simulink model "Alu8Bit"  (R2014a)
settings: Solver=ode45  StartTime=0.0  StopTime=10.0  RelTol=1e-3
libraries: hdlsllib x104
(part 1 of 5)
settings Model: Creator=you.r  LastModifiedBy=you.r
settings OptimizationCC: BlockReduction=off  ConditionallyExecuteInputs=off  InlineParams=on
settings DebuggingCC: AlgebraicLoopMsg=error
settings HardwareCC: ProdHWDeviceType=ASIC/FPGA->ASIC/FPGA  ProdEqTarget=off

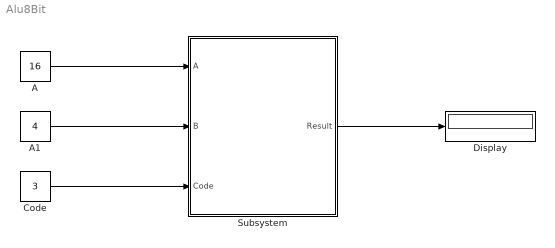
== system Alu8Bit ==
  A : Constant  Value=16  OutDataTypeStr=uint8  SampleTime=1
  A1 : Constant  Value=4  OutDataTypeStr=uint8  SampleTime=1
  Code : Constant  Value=3  OutDataTypeStr=uint8  SampleTime=1
  Display : Display
  Subsystem : Subsystem  TreatAsAtomicUnit=on
  wires:
  Subsystem/1(Result) -> Display/1
  A/1 -> Subsystem/1(A)
  A1/1 -> Subsystem/2(B)
  Code/1 -> Subsystem/3(Code)

== system Alu8Bit/Subsystem ==
  A : Inport  OutDataTypeStr=uint8  SampleTime=1
  B : Inport  Port=2  OutDataTypeStr=uint8  SampleTime=1
  Code : Inport  Port=3  OutDataTypeStr=uint8  SampleTime=1
  8-bit 4-to-1 MUX : Subsystem
  8-bit Adder : Subsystem
  8-bit Subtractor : Subsystem
  BitwiseAnd : Subsystem
  Multiplier : Subsystem
  Result : Outport
  wires:
  8-bit 4-to-1 MUX/1(y) -> Result/1
  BitwiseAnd/1(y) -> 8-bit 4-to-1 MUX/4(3)
  Multiplier/1(Out1) -> 8-bit 4-to-1 MUX/3(2)
  B/1 -> BitwiseAnd/2(b), Multiplier/2(In2), 8-bit Subtractor/2(In2), 8-bit Adder/2(In2)
  A/1 -> Multiplier/1(In1), BitwiseAnd/1(a), 8-bit Subtractor/1(In1), 8-bit Adder/1(In1)
  8-bit Subtractor/1(Out1) -> 8-bit 4-to-1 MUX/2(1)
  Code/1 -> 8-bit 4-to-1 MUX/5(C)
  8-bit Adder/1(Out1) -> 8-bit 4-to-1 MUX/1(0)

== system Alu8Bit/Subsystem/8-bit 4-to-1 MUX ==
  0 : Inport  OutDataTypeStr=uint8  SampleTime=1
  1 : Inport  Port=2  OutDataTypeStr=uint8  SampleTime=1
  2 : Inport  Port=3  OutDataTypeStr=uint8  SampleTime=1
  3 : Inport  Port=4  OutDataTypeStr=uint8  SampleTime=1
  C : Inport  Port=5  OutDataTypeStr=uint8  SampleTime=1
  Bit Concat : Subsystem
  Subsystem1 : Subsystem
  Subsystem2 : Subsystem
  Subsystem3 : Subsystem
  Subsystem4 : Subsystem
  Subsystem5 : Subsystem
  Subsystem6 : Subsystem
  Subsystem7 : Subsystem
  Subsystem8 : Subsystem
  X Slicer1 : Subsystem
  X Slicer2 : Subsystem
  X Slicer3 : Subsystem
  X Slicer4 : Subsystem
  X Slicer5 : Subsystem
  y : Outport  SampleTime=1
  wires:
  X Slicer1/4(Y3) -> Subsystem3/4(I2)
  1/1 -> X Slicer1/1(X)
  X Slicer3/2(Y1) -> Subsystem1/5(I3)
  X Slicer4/4(Y3) -> Subsystem3/6(I4)
  X Slicer1/1(Y0) -> Subsystem8/4(I2)
  X Slicer1/2(Y1) -> Subsystem1/4(I2)
  X Slicer2/3(Y2) -> Subsystem2/3(I1)
  X Slicer5/2(C2) -> Subsystem2/1(C2), Subsystem1/1(C2), Subsystem8/1(C2), Subsystem3/1(C2), Subsystem5/1(C2), Subsystem6/1(C2), Subsystem7/1(C2), Subsystem4/1(C2)
  X Slicer1/3(Y2) -> Subsystem2/4(I2)
  X Slicer3/7(Y6) -> Subsystem6/5(I3)
  X Slicer2/2(Y1) -> Subsystem1/3(I1)
  X Slicer5/1(C1) -> Subsystem2/2(C1), Subsystem1/2(C1), Subsystem8/2(C1), Subsystem3/2(C1), Subsystem4/2(C1), Subsystem5/2(C1), Subsystem7/2(C1), Subsystem6/2(C1)
  X Slicer4/1(Y0) -> Subsystem8/6(I4)
  0/1 -> X Slicer2/1(X)
  X Slicer3/1(Y0) -> Subsystem8/5(I3)
  X Slicer1/8(Y7) -> Subsystem7/4(I2)
  X Slicer1/5(Y4) -> Subsystem4/4(I2)
  X Slicer3/6(Y5) -> Subsystem5/5(I3)
  X Slicer4/2(Y1) -> Subsystem1/6(I4)
  X Slicer2/6(Y5) -> Subsystem5/3(I1)
  X Slicer4/6(Y5) -> Subsystem5/6(I4)
  X Slicer1/6(Y5) -> Subsystem5/4(I2)
  X Slicer2/1(Y0) -> Subsystem8/3(I1)
  X Slicer4/3(Y2) -> Subsystem2/6(I4)
  X Slicer2/5(Y4) -> Subsystem4/3(I1)
  2/1 -> X Slicer3/1(X)
  3/1 -> X Slicer4/1(X)
  X Slicer1/7(Y6) -> Subsystem6/4(I2)
  Bit Concat/1(Out1) -> y/1
  X Slicer4/7(Y6) -> Subsystem6/6(I4)
  X Slicer3/5(Y4) -> Subsystem4/5(I3)
  X Slicer2/7(Y6) -> Subsystem6/3(I1)
  C/1 -> X Slicer5/1(X)
  X Slicer2/4(Y3) -> Subsystem3/3(I1)
  X Slicer4/5(Y4) -> Subsystem4/6(I4)
  X Slicer3/4(Y3) -> Subsystem3/5(I3)
  X Slicer4/8(Y7) -> Subsystem7/6(I4)
  X Slicer3/8(Y7) -> Subsystem7/5(I3)
  Subsystem2/1(Out) -> Bit Concat/6(In6)
  Subsystem1/1(Out) -> Bit Concat/7(In7)
  Subsystem8/1(Out) -> Bit Concat/8(In8)
  Subsystem3/1(Out) -> Bit Concat/5(In5)
  Subsystem6/1(Out) -> Bit Concat/2(In2)
  Subsystem4/1(Out) -> Bit Concat/4(In4)
  Subsystem5/1(Out) -> Bit Concat/3(In3)
  Subsystem7/1(Out) -> Bit Concat/1(In1)
  X Slicer2/8(Y7) -> Subsystem7/3(I1)
  X Slicer3/3(Y2) -> Subsystem2/5(I3)

== system Alu8Bit/Subsystem/8-bit Adder ==
  In1 : Inport
  In2 : Inport  Port=2
  8-bit Adder : Subsystem
  Bit Concat : Subsystem
  Both Negative : Logic  AllPortsSameDT=off  OutDataTypeStr=boolean
  Both Positive : Logic  AllPortsSameDT=off  OutDataTypeStr=boolean
  "If both conditions true, overflow" : Logic  AllPortsSameDT=off  OutDataTypeStr=boolean
  "If both conditions true, overflow1" : Logic  AllPortsSameDT=off  OutDataTypeStr=boolean
  MSB Not High : Logic  Operator=NOT  AllPortsSameDT=off  OutDataTypeStr=boolean
  Negative Or MSB HIgh : Logic  Operator=XOR  AllPortsSameDT=off  OutDataTypeStr=boolean
  Positive A : Logic  Operator=NOT  AllPortsSameDT=off  OutDataTypeStr=boolean
  Positive B : Logic  Operator=NOT  AllPortsSameDT=off  OutDataTypeStr=boolean
  Positive or MSB not high : Logic  Operator=XOR  AllPortsSameDT=off  OutDataTypeStr=boolean
  Subtract : Constant  Value=0  OutDataTypeStr=boolean  SampleTime=1
  X Slicer : Subsystem
  X Slicer1 : Subsystem
  Xor : Logic  Operator=XOR  AllPortsSameDT=off  OutDataTypeStr=boolean
  Xor1 : Logic  Operator=XOR  AllPortsSameDT=off  OutDataTypeStr=boolean
  Out1 : Outport
  Out2 : Outport  Port=2
  wires:
  Bit Concat/1(Out1) -> Out1/1
  In1/1 -> X Slicer/1(X)
  In2/1 -> X Slicer1/1(X)
  8-bit Adder/8(Out8) -> Negative Or MSB HIgh/1, MSB Not High/1, Bit Concat/1(In1)
  8-bit Adder/7(Out7) -> Bit Concat/2(In2)
  8-bit Adder/6(Out6) -> Bit Concat/3(In3)
  8-bit Adder/5(Out5) -> Bit Concat/4(In4)
  8-bit Adder/4(Out4) -> Bit Concat/5(In5)
  8-bit Adder/3(Out3) -> Bit Concat/6(In6)
  8-bit Adder/2(Out2) -> Bit Concat/7(In7)
  8-bit Adder/1(Out1) -> Bit Concat/8(In8)
  X Slicer/1(Y0) -> 8-bit Adder/1(A1)
  X Slicer/2(Y1) -> 8-bit Adder/3(A2)
  X Slicer/3(Y2) -> 8-bit Adder/4(A3)
  X Slicer/4(Y3) -> 8-bit Adder/5(A4)
  X Slicer/5(Y4) -> 8-bit Adder/9(A5)
  X Slicer/6(Y5) -> 8-bit Adder/6(A6)
  X Slicer/7(Y6) -> 8-bit Adder/7(A7)
  X Slicer1/1(Y0) -> 8-bit Adder/2(B1)
  X Slicer1/2(Y1) -> 8-bit Adder/10(B2)
  X Slicer1/3(Y2) -> 8-bit Adder/11(B3)
  X Slicer1/4(Y3) -> 8-bit Adder/12(B4)
  X Slicer1/5(Y4) -> 8-bit Adder/16(B5)
  X Slicer1/6(Y5) -> 8-bit Adder/13(B6)
  X Slicer1/7(Y6) -> 8-bit Adder/14(B7)
  X Slicer1/8(Y7) -> Xor1/1, 8-bit Adder/15(B8)
  Both Negative/1 -> "If both conditions true, overflow"/2, Negative Or MSB HIgh/2
  Negative Or MSB HIgh/1 -> "If both conditions true, overflow"/1
  X Slicer/8(Y7) -> Positive A/1, Both Negative/1, 8-bit Adder/8(A8)
  Positive A/1 -> Both Positive/1
  Positive B/1 -> Both Positive/2
  Both Positive/1 -> "If both conditions true, overflow1"/1, Positive or MSB not high/1
  MSB Not High/1 -> Positive or MSB not high/2
  Positive or MSB not high/1 -> "If both conditions true, overflow1"/2
  Xor/1 -> Out2/1
  "If both conditions true, overflow1"/1 -> Xor/2
  "If both conditions true, overflow"/1 -> Xor/1
  Subtract/1 -> Xor1/2, 8-bit Adder/17(Subtraction?)
  Xor1/1 -> Positive B/1, Both Negative/2

== system Alu8Bit/Subsystem/8-bit Subtractor ==
  In1 : Inport
  In2 : Inport  Port=2
  8-bit Adder : Subsystem
  Bit Concat : Subsystem
  Both Negative : Logic  AllPortsSameDT=off  OutDataTypeStr=boolean
  Both Positive : Logic  AllPortsSameDT=off  OutDataTypeStr=boolean
  "If both conditions true, overflow" : Logic  AllPortsSameDT=off  OutDataTypeStr=boolean
  "If both conditions true, overflow1" : Logic  AllPortsSameDT=off  OutDataTypeStr=boolean
  MSB Not High : Logic  Operator=NOT  AllPortsSameDT=off  OutDataTypeStr=boolean
  Negative Or MSB HIgh : Logic  Operator=XOR  AllPortsSameDT=off  OutDataTypeStr=boolean
  Positive A : Logic  Operator=NOT  AllPortsSameDT=off  OutDataTypeStr=boolean
  Positive B : Logic  Operator=NOT  AllPortsSameDT=off  OutDataTypeStr=boolean
  Positive or MSB not high : Logic  Operator=XOR  AllPortsSameDT=off  OutDataTypeStr=boolean
  Subtract : Constant  OutDataTypeStr=boolean  SampleTime=1
  X Slicer : Subsystem
  X Slicer1 : Subsystem
  Xor : Logic  Operator=XOR  AllPortsSameDT=off  OutDataTypeStr=boolean
  Xor1 : Logic  Operator=XOR  AllPortsSameDT=off  OutDataTypeStr=boolean
  Out1 : Outport
  Out2 : Outport  Port=2
  wires:
  Bit Concat/1(Out1) -> Out1/1
  In1/1 -> X Slicer/1(X)
  In2/1 -> X Slicer1/1(X)
  8-bit Adder/8(Out8) -> Negative Or MSB HIgh/1, MSB Not High/1, Bit Concat/1(In1)
  8-bit Adder/7(Out7) -> Bit Concat/2(In2)
  8-bit Adder/6(Out6) -> Bit Concat/3(In3)
  8-bit Adder/5(Out5) -> Bit Concat/4(In4)
  8-bit Adder/4(Out4) -> Bit Concat/5(In5)
  8-bit Adder/3(Out3) -> Bit Concat/6(In6)
  8-bit Adder/2(Out2) -> Bit Concat/7(In7)
  8-bit Adder/1(Out1) -> Bit Concat/8(In8)
  X Slicer/1(Y0) -> 8-bit Adder/1(A1)
  X Slicer/2(Y1) -> 8-bit Adder/3(A2)
  X Slicer/3(Y2) -> 8-bit Adder/4(A3)
  X Slicer/4(Y3) -> 8-bit Adder/5(A4)
  X Slicer/5(Y4) -> 8-bit Adder/9(A5)
  X Slicer/6(Y5) -> 8-bit Adder/6(A6)
  X Slicer/7(Y6) -> 8-bit Adder/7(A7)
  X Slicer1/1(Y0) -> 8-bit Adder/2(B1)
  X Slicer1/2(Y1) -> 8-bit Adder/10(B2)
  X Slicer1/3(Y2) -> 8-bit Adder/11(B3)
  X Slicer1/4(Y3) -> 8-bit Adder/12(B4)
  X Slicer1/5(Y4) -> 8-bit Adder/16(B5)
  X Slicer1/6(Y5) -> 8-bit Adder/13(B6)
  X Slicer1/7(Y6) -> 8-bit Adder/14(B7)
  X Slicer1/8(Y7) -> Xor1/1, 8-bit Adder/15(B8)
  Both Negative/1 -> "If both conditions true, overflow"/2, Negative Or MSB HIgh/2
  Negative Or MSB HIgh/1 -> "If both conditions true, overflow"/1
  X Slicer/8(Y7) -> Positive A/1, Both Negative/1, 8-bit Adder/8(A8)
  Positive A/1 -> Both Positive/1
  Positive B/1 -> Both Positive/2
  Both Positive/1 -> "If both conditions true, overflow1"/1, Positive or MSB not high/1
  MSB Not High/1 -> Positive or MSB not high/2
  Positive or MSB not high/1 -> "If both conditions true, overflow1"/2
  Xor/1 -> Out2/1
  "If both conditions true, overflow1"/1 -> Xor/2
  "If both conditions true, overflow"/1 -> Xor/1
  Subtract/1 -> Xor1/2, 8-bit Adder/17(Subtraction?)
  Xor1/1 -> Positive B/1, Both Negative/2

== system Alu8Bit/Subsystem/BitwiseAnd ==
  a : Inport  OutDataTypeStr=uint8  SampleTime=1
  b : Inport  Port=2  OutDataTypeStr=uint8  SampleTime=1
  Bit Concat : Subsystem
  Logical Operator{,1..7} (8 alike) : Logic  IconShape=distinctive  AllPortsSameDT=off  OutDataTypeStr=boolean  SampleTime=1
  X Slicer1 : Subsystem
  X Slicer2 : Subsystem
  y : Outport  SampleTime=1
  wires:
  b/1 -> X Slicer1/1(X)
  a/1 -> X Slicer2/1(X)
  Logical Operator2/1 -> Bit Concat/6(In6)
  Logical Operator4/1 -> Bit Concat/4(In4)
  Logical Operator7/1 -> Bit Concat/1(In1)
  Logical Operator/1 -> Bit Concat/8(In8)
  Logical Operator1/1 -> Bit Concat/7(In7)
  Logical Operator6/1 -> Bit Concat/2(In2)
  Logical Operator5/1 -> Bit Concat/3(In3)
  Logical Operator3/1 -> Bit Concat/5(In5)
  X Slicer1/8(Y7) -> Logical Operator7/2
  X Slicer1/5(Y4) -> Logical Operator4/2
  X Slicer2/4(Y3) -> Logical Operator3/1
  X Slicer2/8(Y7) -> Logical Operator7/1
  X Slicer2/3(Y2) -> Logical Operator2/1
  X Slicer2/6(Y5) -> Logical Operator5/1
  X Slicer2/2(Y1) -> Logical Operator1/1
  X Slicer1/3(Y2) -> Logical Operator2/2
  X Slicer1/2(Y1) -> Logical Operator1/2
  X Slicer1/7(Y6) -> Logical Operator6/2
  X Slicer2/7(Y6) -> Logical Operator6/1
  X Slicer2/5(Y4) -> Logical Operator4/1
  X Slicer1/1(Y0) -> Logical Operator/2
  X Slicer2/1(Y0) -> Logical Operator/1
  X Slicer1/6(Y5) -> Logical Operator5/2
  X Slicer1/4(Y3) -> Logical Operator3/2
  Bit Concat/1(Out1) -> y/1

== system Alu8Bit/Subsystem/Multiplier ==
  In1 : Inport  OutDataTypeStr=uint8
  In2 : Inport  Port=2  OutDataTypeStr=uint8
  Bit Concat : Subsystem
  Multiplier : Subsystem
  X Slicer : Subsystem
  X Slicer1 : Subsystem
  Out1 : Outport
  wires:
  In2/1 -> X Slicer1/1(X)
  In1/1 -> X Slicer/1(X)
  Bit Concat/1(Out1) -> Out1/1
  Multiplier/1(P0) -> Bit Concat/16(In16)
  Multiplier/2(P1) -> Bit Concat/15(In15)
  Multiplier/3(P2) -> Bit Concat/14(In14)
  Multiplier/4(P3) -> Bit Concat/13(In13)
  Multiplier/5(P4) -> Bit Concat/12(In12)
  Multiplier/6(P5) -> Bit Concat/11(In11)
  Multiplier/7(P6) -> Bit Concat/10(In10)
  Multiplier/8(P7) -> Bit Concat/9(In9)
  Multiplier/9(P15) -> Bit Concat/1(In1)
  Multiplier/10(P14) -> Bit Concat/2(In2)
  Multiplier/11(P13) -> Bit Concat/3(In3)
  Multiplier/12(P12) -> Bit Concat/4(In4)
  Multiplier/13(P11) -> Bit Concat/5(In5)
  Multiplier/14(P10) -> Bit Concat/6(In6)
  Multiplier/15(P9) -> Bit Concat/7(In7)
  Multiplier/16(P8) -> Bit Concat/8(In8)
  X Slicer/1(Y0) -> Multiplier/8(A0)
  X Slicer/2(Y1) -> Multiplier/7(A1)
  X Slicer/3(Y2) -> Multiplier/6(A2)
  X Slicer/4(Y3) -> Multiplier/5(A3)
  X Slicer/5(Y4) -> Multiplier/4(A4)
  X Slicer/6(Y5) -> Multiplier/3(A5)
  X Slicer/7(Y6) -> Multiplier/2(A6)
  X Slicer/8(Y7) -> Multiplier/1(A7)
  X Slicer1/1(Y0) -> Multiplier/9(B0)
  X Slicer1/2(Y1) -> Multiplier/10(B1)
  X Slicer1/3(Y2) -> Multiplier/11(B2)
  X Slicer1/4(Y3) -> Multiplier/12(B3)
  X Slicer1/5(Y4) -> Multiplier/13(B4)
  X Slicer1/6(Y5) -> Multiplier/14(B5)
  X Slicer1/7(Y6) -> Multiplier/15(B6)
  X Slicer1/8(Y7) -> Multiplier/16(B7)

== system Alu8Bit/Subsystem/8-bit 4-to-1 MUX/Bit Concat ==
  In1 : Inport
  In2 : Inport  Port=2
  In3 : Inport  Port=3
  In4 : Inport  Port=4
  In5 : Inport  Port=5
  In6 : Inport  Port=6
  In7 : Inport  Port=7
  In8 : Inport  Port=8
  Bit Concat : hdlsllib/HDL Operations/Bit Concat  numInputs=8
  Data Type Conversion : DataTypeConversion  OutDataTypeStr=uint8
  Out1 : Outport
  wires:
  Data Type Conversion/1 -> Out1/1
  Bit Concat/1 -> Data Type Conversion/1
  In7/1 -> Bit Concat/7
  In1/1 -> Bit Concat/1
  In8/1 -> Bit Concat/8
  In6/1 -> Bit Concat/6
  In2/1 -> Bit Concat/2
  In5/1 -> Bit Concat/5
  In3/1 -> Bit Concat/3
  In4/1 -> Bit Concat/4

== system Alu8Bit/Subsystem/8-bit 4-to-1 MUX/Subsystem1 ==
  C2 : Inport
  C1 : Inport  Port=2
  I1 : Inport  Port=3
  I2 : Inport  Port=4
  I3 : Inport  Port=5
  I4 : Inport  Port=6
  Logical Operator{,1..5,7,9} (8 alike) : Logic  IconShape=distinctive  AllPortsSameDT=off  OutDataTypeStr=boolean
  Logical Operator10 : Logic  Operator=NOT  IconShape=distinctive  AllPortsSameDT=off  OutDataTypeStr=boolean
  Logical Operator6 : Logic  Operator=OR  Inputs=4  IconShape=distinctive  AllPortsSameDT=off  OutDataTypeStr=boolean
  Logical Operator8 : Logic  Operator=NOT  IconShape=distinctive  AllPortsSameDT=off  OutDataTypeStr=boolean
  Out : Outport
  wires:
  I1/1 -> Logical Operator2/1
  I3/1 -> Logical Operator5/1
  Logical Operator4/1 -> Logical Operator6/4
  Logical Operator3/1 -> Logical Operator6/2
  C1/1 -> Logical Operator10/1, Logical Operator/2, Logical Operator7/2
  C2/1 -> Logical Operator9/2, Logical Operator/1, Logical Operator8/1
  Logical Operator10/1 -> Logical Operator1/1, Logical Operator9/1
  Logical Operator/1 -> Logical Operator4/2
  Logical Operator7/1 -> Logical Operator3/2
  I2/1 -> Logical Operator3/1
  Logical Operator2/1 -> Logical Operator6/1
  Logical Operator9/1 -> Logical Operator5/2
  I4/1 -> Logical Operator4/1
  Logical Operator5/1 -> Logical Operator6/3
  Logical Operator6/1 -> Out/1
  Logical Operator8/1 -> Logical Operator1/2, Logical Operator7/1
  Logical Operator1/1 -> Logical Operator2/2

== system Alu8Bit/Subsystem/8-bit 4-to-1 MUX/Subsystem2 ==
  C2 : Inport
  C1 : Inport  Port=2
  I1 : Inport  Port=3
  I2 : Inport  Port=4
  I3 : Inport  Port=5
  I4 : Inport  Port=6
  Logical Operator{,1..5,7,9} (8 alike) : Logic  IconShape=distinctive  AllPortsSameDT=off  OutDataTypeStr=boolean
  Logical Operator10 : Logic  Operator=NOT  IconShape=distinctive  AllPortsSameDT=off  OutDataTypeStr=boolean
  Logical Operator6 : Logic  Operator=OR  Inputs=4  IconShape=distinctive  AllPortsSameDT=off  OutDataTypeStr=boolean
  Logical Operator8 : Logic  Operator=NOT  IconShape=distinctive  AllPortsSameDT=off  OutDataTypeStr=boolean
  Out : Outport
  wires:
  I1/1 -> Logical Operator2/1
  I3/1 -> Logical Operator5/1
  Logical Operator4/1 -> Logical Operator6/4
  Logical Operator3/1 -> Logical Operator6/2
  C1/1 -> Logical Operator10/1, Logical Operator/2, Logical Operator7/2
  C2/1 -> Logical Operator9/2, Logical Operator/1, Logical Operator8/1
  Logical Operator10/1 -> Logical Operator1/1, Logical Operator9/1
  Logical Operator/1 -> Logical Operator4/2
  Logical Operator7/1 -> Logical Operator3/2
  I2/1 -> Logical Operator3/1
  Logical Operator2/1 -> Logical Operator6/1
  Logical Operator9/1 -> Logical Operator5/2
  I4/1 -> Logical Operator4/1
  Logical Operator5/1 -> Logical Operator6/3
  Logical Operator6/1 -> Out/1
  Logical Operator8/1 -> Logical Operator1/2, Logical Operator7/1
  Logical Operator1/1 -> Logical Operator2/2

== system Alu8Bit/Subsystem/8-bit 4-to-1 MUX/Subsystem3 ==
  C2 : Inport
  C1 : Inport  Port=2
  I1 : Inport  Port=3
  I2 : Inport  Port=4
  I3 : Inport  Port=5
  I4 : Inport  Port=6
  Logical Operator{,1..5,7,9} (8 alike) : Logic  IconShape=distinctive  AllPortsSameDT=off  OutDataTypeStr=boolean
  Logical Operator10 : Logic  Operator=NOT  IconShape=distinctive  AllPortsSameDT=off  OutDataTypeStr=boolean
  Logical Operator6 : Logic  Operator=OR  Inputs=4  IconShape=distinctive  AllPortsSameDT=off  OutDataTypeStr=boolean
  Logical Operator8 : Logic  Operator=NOT  IconShape=distinctive  AllPortsSameDT=off  OutDataTypeStr=boolean
  Out : Outport
  wires:
  I1/1 -> Logical Operator2/1
  I3/1 -> Logical Operator5/1
  Logical Operator4/1 -> Logical Operator6/4
  Logical Operator3/1 -> Logical Operator6/2
  C1/1 -> Logical Operator10/1, Logical Operator/2, Logical Operator7/2
  C2/1 -> Logical Operator9/2, Logical Operator/1, Logical Operator8/1
  Logical Operator10/1 -> Logical Operator1/1, Logical Operator9/1
  Logical Operator/1 -> Logical Operator4/2
  Logical Operator7/1 -> Logical Operator3/2
  I2/1 -> Logical Operator3/1
  Logical Operator2/1 -> Logical Operator6/1
  Logical Operator9/1 -> Logical Operator5/2
  I4/1 -> Logical Operator4/1
  Logical Operator5/1 -> Logical Operator6/3
  Logical Operator6/1 -> Out/1
  Logical Operator8/1 -> Logical Operator1/2, Logical Operator7/1
  Logical Operator1/1 -> Logical Operator2/2

== system Alu8Bit/Subsystem/8-bit 4-to-1 MUX/Subsystem4 ==
  C2 : Inport
  C1 : Inport  Port=2
  I1 : Inport  Port=3
  I2 : Inport  Port=4
  I3 : Inport  Port=5
  I4 : Inport  Port=6
  Logical Operator{,1..5,7,9} (8 alike) : Logic  IconShape=distinctive  AllPortsSameDT=off  OutDataTypeStr=boolean
  Logical Operator10 : Logic  Operator=NOT  IconShape=distinctive  AllPortsSameDT=off  OutDataTypeStr=boolean
  Logical Operator6 : Logic  Operator=OR  Inputs=4  IconShape=distinctive  AllPortsSameDT=off  OutDataTypeStr=boolean
  Logical Operator8 : Logic  Operator=NOT  IconShape=distinctive  AllPortsSameDT=off  OutDataTypeStr=boolean
  Out : Outport
  wires:
  I1/1 -> Logical Operator2/1
  I3/1 -> Logical Operator5/1
  Logical Operator4/1 -> Logical Operator6/4
  Logical Operator3/1 -> Logical Operator6/2
  C1/1 -> Logical Operator10/1, Logical Operator/2, Logical Operator7/2
  C2/1 -> Logical Operator9/2, Logical Operator/1, Logical Operator8/1
  Logical Operator10/1 -> Logical Operator1/1, Logical Operator9/1
  Logical Operator/1 -> Logical Operator4/2
  Logical Operator7/1 -> Logical Operator3/2
  I2/1 -> Logical Operator3/1
  Logical Operator2/1 -> Logical Operator6/1
  Logical Operator9/1 -> Logical Operator5/2
  I4/1 -> Logical Operator4/1
  Logical Operator5/1 -> Logical Operator6/3
  Logical Operator6/1 -> Out/1
  Logical Operator8/1 -> Logical Operator1/2, Logical Operator7/1
  Logical Operator1/1 -> Logical Operator2/2

== system Alu8Bit/Subsystem/8-bit 4-to-1 MUX/Subsystem5 ==
  C2 : Inport
  C1 : Inport  Port=2
  I1 : Inport  Port=3
  I2 : Inport  Port=4
  I3 : Inport  Port=5
  I4 : Inport  Port=6
  Logical Operator{,1..5,7,9} (8 alike) : Logic  IconShape=distinctive  AllPortsSameDT=off  OutDataTypeStr=boolean
  Logical Operator10 : Logic  Operator=NOT  IconShape=distinctive  AllPortsSameDT=off  OutDataTypeStr=boolean
  Logical Operator6 : Logic  Operator=OR  Inputs=4  IconShape=distinctive  AllPortsSameDT=off  OutDataTypeStr=boolean
  Logical Operator8 : Logic  Operator=NOT  IconShape=distinctive  AllPortsSameDT=off  OutDataTypeStr=boolean
  Out : Outport
  wires:
  I1/1 -> Logical Operator2/1
  I3/1 -> Logical Operator5/1
  Logical Operator4/1 -> Logical Operator6/4
  Logical Operator3/1 -> Logical Operator6/2
  C1/1 -> Logical Operator10/1, Logical Operator/2, Logical Operator7/2
  C2/1 -> Logical Operator9/2, Logical Operator/1, Logical Operator8/1
  Logical Operator10/1 -> Logical Operator1/1, Logical Operator9/1
  Logical Operator/1 -> Logical Operator4/2
  Logical Operator7/1 -> Logical Operator3/2
  I2/1 -> Logical Operator3/1
  Logical Operator2/1 -> Logical Operator6/1
  Logical Operator9/1 -> Logical Operator5/2
  I4/1 -> Logical Operator4/1
  Logical Operator5/1 -> Logical Operator6/3
  Logical Operator6/1 -> Out/1
  Logical Operator8/1 -> Logical Operator1/2, Logical Operator7/1
  Logical Operator1/1 -> Logical Operator2/2

== system Alu8Bit/Subsystem/8-bit 4-to-1 MUX/Subsystem6 ==
  C2 : Inport
  C1 : Inport  Port=2
  I1 : Inport  Port=3
  I2 : Inport  Port=4
  I3 : Inport  Port=5
  I4 : Inport  Port=6
  Logical Operator{,1..5,7,9} (8 alike) : Logic  IconShape=distinctive  AllPortsSameDT=off  OutDataTypeStr=boolean
  Logical Operator10 : Logic  Operator=NOT  IconShape=distinctive  AllPortsSameDT=off  OutDataTypeStr=boolean
  Logical Operator6 : Logic  Operator=OR  Inputs=4  IconShape=distinctive  AllPortsSameDT=off  OutDataTypeStr=boolean
  Logical Operator8 : Logic  Operator=NOT  IconShape=distinctive  AllPortsSameDT=off  OutDataTypeStr=boolean
  Out : Outport
  wires:
  I1/1 -> Logical Operator2/1
  I3/1 -> Logical Operator5/1
  Logical Operator4/1 -> Logical Operator6/4
  Logical Operator3/1 -> Logical Operator6/2
  C1/1 -> Logical Operator10/1, Logical Operator/2, Logical Operator7/2
  C2/1 -> Logical Operator9/2, Logical Operator/1, Logical Operator8/1
  Logical Operator10/1 -> Logical Operator1/1, Logical Operator9/1
  Logical Operator/1 -> Logical Operator4/2
  Logical Operator7/1 -> Logical Operator3/2
  I2/1 -> Logical Operator3/1
  Logical Operator2/1 -> Logical Operator6/1
  Logical Operator9/1 -> Logical Operator5/2
  I4/1 -> Logical Operator4/1
  Logical Operator5/1 -> Logical Operator6/3
  Logical Operator6/1 -> Out/1
  Logical Operator8/1 -> Logical Operator1/2, Logical Operator7/1
  Logical Operator1/1 -> Logical Operator2/2

== system Alu8Bit/Subsystem/8-bit 4-to-1 MUX/Subsystem7 ==
  C2 : Inport
  C1 : Inport  Port=2
  I1 : Inport  Port=3
  I2 : Inport  Port=4
  I3 : Inport  Port=5
  I4 : Inport  Port=6
  Logical Operator{,1..5,7,9} (8 alike) : Logic  IconShape=distinctive  AllPortsSameDT=off  OutDataTypeStr=boolean
  Logical Operator10 : Logic  Operator=NOT  IconShape=distinctive  AllPortsSameDT=off  OutDataTypeStr=boolean
  Logical Operator6 : Logic  Operator=OR  Inputs=4  IconShape=distinctive  AllPortsSameDT=off  OutDataTypeStr=boolean
  Logical Operator8 : Logic  Operator=NOT  IconShape=distinctive  AllPortsSameDT=off  OutDataTypeStr=boolean
  Out : Outport
  wires:
  I1/1 -> Logical Operator2/1
  I3/1 -> Logical Operator5/1
  Logical Operator4/1 -> Logical Operator6/4
  Logical Operator3/1 -> Logical Operator6/2
  C1/1 -> Logical Operator10/1, Logical Operator/2, Logical Operator7/2
  C2/1 -> Logical Operator9/2, Logical Operator/1, Logical Operator8/1
  Logical Operator10/1 -> Logical Operator1/1, Logical Operator9/1
  Logical Operator/1 -> Logical Operator4/2
  Logical Operator7/1 -> Logical Operator3/2
  I2/1 -> Logical Operator3/1
  Logical Operator2/1 -> Logical Operator6/1
  Logical Operator9/1 -> Logical Operator5/2
  I4/1 -> Logical Operator4/1
  Logical Operator5/1 -> Logical Operator6/3
  Logical Operator6/1 -> Out/1
  Logical Operator8/1 -> Logical Operator1/2, Logical Operator7/1
  Logical Operator1/1 -> Logical Operator2/2

== system Alu8Bit/Subsystem/8-bit 4-to-1 MUX/Subsystem8 ==
  C2 : Inport
  C1 : Inport  Port=2
  I1 : Inport  Port=3
  I2 : Inport  Port=4
  I3 : Inport  Port=5
  I4 : Inport  Port=6
  Logical Operator{,1..5,7,9} (8 alike) : Logic  IconShape=distinctive  AllPortsSameDT=off  OutDataTypeStr=boolean
  Logical Operator10 : Logic  Operator=NOT  IconShape=distinctive  AllPortsSameDT=off  OutDataTypeStr=boolean
  Logical Operator6 : Logic  Operator=OR  Inputs=4  IconShape=distinctive  AllPortsSameDT=off  OutDataTypeStr=boolean
  Logical Operator8 : Logic  Operator=NOT  IconShape=distinctive  AllPortsSameDT=off  OutDataTypeStr=boolean
  Out : Outport
  wires:
  I1/1 -> Logical Operator2/1
  I3/1 -> Logical Operator5/1
  Logical Operator4/1 -> Logical Operator6/4
  Logical Operator3/1 -> Logical Operator6/2
  C1/1 -> Logical Operator10/1, Logical Operator/2, Logical Operator7/2
  C2/1 -> Logical Operator9/2, Logical Operator/1, Logical Operator8/1
  Logical Operator10/1 -> Logical Operator1/1, Logical Operator9/1
  Logical Operator/1 -> Logical Operator4/2
  Logical Operator7/1 -> Logical Operator3/2
  I2/1 -> Logical Operator3/1
  Logical Operator2/1 -> Logical Operator6/1
  Logical Operator9/1 -> Logical Operator5/2
  I4/1 -> Logical Operator4/1
  Logical Operator5/1 -> Logical Operator6/3
  Logical Operator6/1 -> Out/1
  Logical Operator8/1 -> Logical Operator1/2, Logical Operator7/1
  Logical Operator1/1 -> Logical Operator2/2

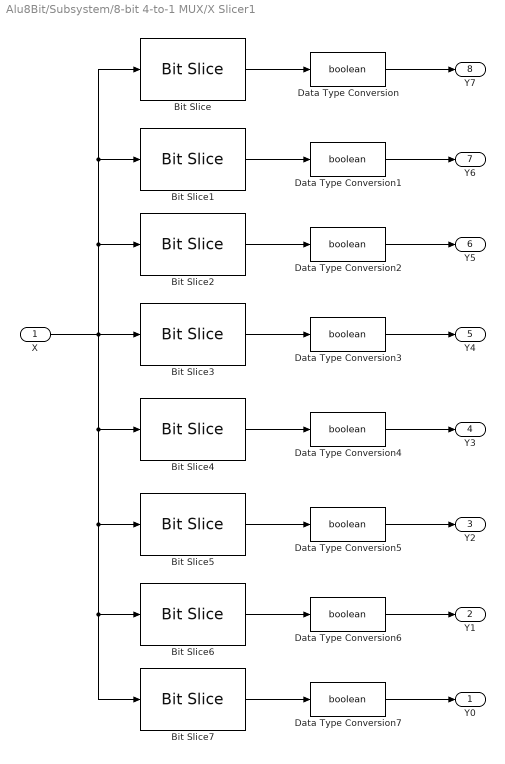
== system Alu8Bit/Subsystem/8-bit 4-to-1 MUX/X Slicer1 ==
  X : Inport  OutDataTypeStr=uint8  SampleTime=1
  Bit Slice : hdlsllib/HDL Operations/Bit Slice  lidx=7  ridx=7
  Bit Slice1 : hdlsllib/HDL Operations/Bit Slice  lidx=6  ridx=6
  Bit Slice2 : hdlsllib/HDL Operations/Bit Slice  lidx=5  ridx=5
  Bit Slice3 : hdlsllib/HDL Operations/Bit Slice  lidx=4  ridx=4
  Bit Slice4 : hdlsllib/HDL Operations/Bit Slice  lidx=3  ridx=3
  Bit Slice5 : hdlsllib/HDL Operations/Bit Slice  lidx=2  ridx=2
  Bit Slice6 : hdlsllib/HDL Operations/Bit Slice  lidx=1  ridx=1
  Bit Slice7 : hdlsllib/HDL Operations/Bit Slice  lidx=0  ridx=0
  Data Type Conversion{,1..7} (8 alike) : DataTypeConversion  OutDataTypeStr=boolean
  Y0 : Outport  OutDataTypeStr=boolean  SampleTime=1
  Y1 : Outport  Port=2  OutDataTypeStr=boolean  SampleTime=1
  Y2 : Outport  Port=3  OutDataTypeStr=boolean  SampleTime=1
  Y3 : Outport  Port=4  OutDataTypeStr=boolean  SampleTime=1
  Y4 : Outport  Port=5  OutDataTypeStr=boolean  SampleTime=1
  Y5 : Outport  Port=6  OutDataTypeStr=boolean  SampleTime=1
  Y6 : Outport  Port=7  OutDataTypeStr=boolean  SampleTime=1
  Y7 : Outport  Port=8  OutDataTypeStr=boolean  SampleTime=1
  wires:
  X/1 -> Bit Slice4/1, Bit Slice5/1, Bit Slice6/1, Bit Slice7/1, Bit Slice3/1, Bit Slice2/1, Bit Slice1/1, Bit Slice/1
  Data Type Conversion/1 -> Y7/1
  Data Type Conversion1/1 -> Y6/1
  Bit Slice2/1 -> Data Type Conversion2/1
  Bit Slice3/1 -> Data Type Conversion3/1
  Bit Slice4/1 -> Data Type Conversion4/1
  Data Type Conversion6/1 -> Y1/1
  Bit Slice/1 -> Data Type Conversion/1
  Bit Slice1/1 -> Data Type Conversion1/1
  Bit Slice6/1 -> Data Type Conversion6/1
  Data Type Conversion7/1 -> Y0/1
  Bit Slice7/1 -> Data Type Conversion7/1
  Bit Slice5/1 -> Data Type Conversion5/1
  Data Type Conversion2/1 -> Y5/1
  Data Type Conversion3/1 -> Y4/1
  Data Type Conversion4/1 -> Y3/1
  Data Type Conversion5/1 -> Y2/1

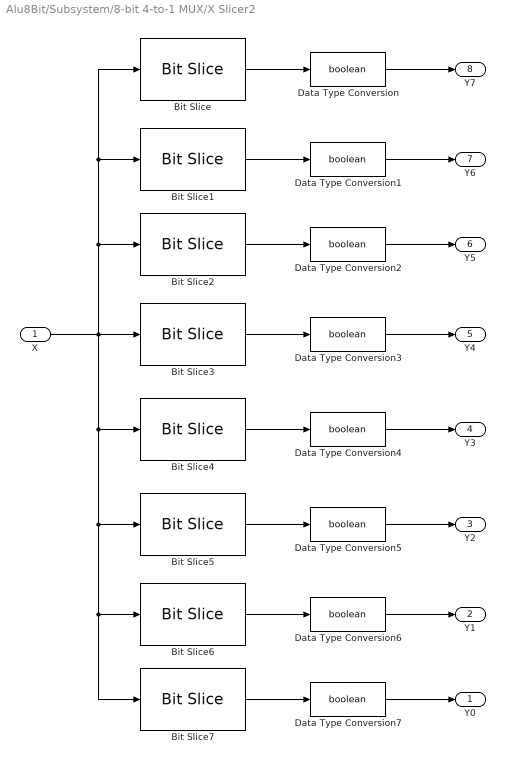
== system Alu8Bit/Subsystem/8-bit 4-to-1 MUX/X Slicer2 ==
  X : Inport  OutDataTypeStr=uint8  SampleTime=1
  Bit Slice : hdlsllib/HDL Operations/Bit Slice  lidx=7  ridx=7
  Bit Slice1 : hdlsllib/HDL Operations/Bit Slice  lidx=6  ridx=6
  Bit Slice2 : hdlsllib/HDL Operations/Bit Slice  lidx=5  ridx=5
  Bit Slice3 : hdlsllib/HDL Operations/Bit Slice  lidx=4  ridx=4
  Bit Slice4 : hdlsllib/HDL Operations/Bit Slice  lidx=3  ridx=3
  Bit Slice5 : hdlsllib/HDL Operations/Bit Slice  lidx=2  ridx=2
  Bit Slice6 : hdlsllib/HDL Operations/Bit Slice  lidx=1  ridx=1
  Bit Slice7 : hdlsllib/HDL Operations/Bit Slice  lidx=0  ridx=0
  Data Type Conversion{,1..7} (8 alike) : DataTypeConversion  OutDataTypeStr=boolean
  Y0 : Outport  OutDataTypeStr=boolean  SampleTime=1
  Y1 : Outport  Port=2  OutDataTypeStr=boolean  SampleTime=1
  Y2 : Outport  Port=3  OutDataTypeStr=boolean  SampleTime=1
  Y3 : Outport  Port=4  OutDataTypeStr=boolean  SampleTime=1
  Y4 : Outport  Port=5  OutDataTypeStr=boolean  SampleTime=1
  Y5 : Outport  Port=6  OutDataTypeStr=boolean  SampleTime=1
  Y6 : Outport  Port=7  OutDataTypeStr=boolean  SampleTime=1
  Y7 : Outport  Port=8  OutDataTypeStr=boolean  SampleTime=1
  wires:
  X/1 -> Bit Slice4/1, Bit Slice5/1, Bit Slice6/1, Bit Slice7/1, Bit Slice3/1, Bit Slice2/1, Bit Slice1/1, Bit Slice/1
  Data Type Conversion/1 -> Y7/1
  Data Type Conversion1/1 -> Y6/1
  Bit Slice2/1 -> Data Type Conversion2/1
  Bit Slice3/1 -> Data Type Conversion3/1
  Bit Slice4/1 -> Data Type Conversion4/1
  Data Type Conversion6/1 -> Y1/1
  Bit Slice/1 -> Data Type Conversion/1
  Bit Slice1/1 -> Data Type Conversion1/1
  Bit Slice6/1 -> Data Type Conversion6/1
  Data Type Conversion7/1 -> Y0/1
  Bit Slice7/1 -> Data Type Conversion7/1
  Bit Slice5/1 -> Data Type Conversion5/1
  Data Type Conversion2/1 -> Y5/1
  Data Type Conversion3/1 -> Y4/1
  Data Type Conversion4/1 -> Y3/1
  Data Type Conversion5/1 -> Y2/1

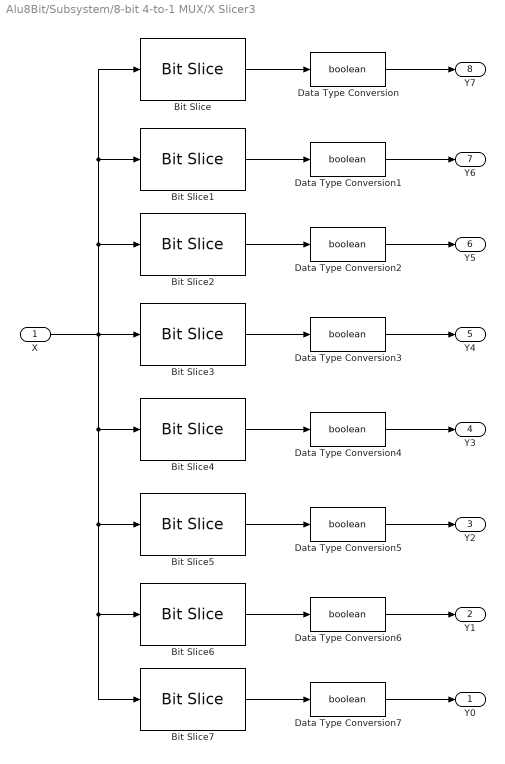
== system Alu8Bit/Subsystem/8-bit 4-to-1 MUX/X Slicer3 ==
  X : Inport  OutDataTypeStr=uint8  SampleTime=1
  Bit Slice : hdlsllib/HDL Operations/Bit Slice  lidx=7  ridx=7
  Bit Slice1 : hdlsllib/HDL Operations/Bit Slice  lidx=6  ridx=6
  Bit Slice2 : hdlsllib/HDL Operations/Bit Slice  lidx=5  ridx=5
  Bit Slice3 : hdlsllib/HDL Operations/Bit Slice  lidx=4  ridx=4
  Bit Slice4 : hdlsllib/HDL Operations/Bit Slice  lidx=3  ridx=3
  Bit Slice5 : hdlsllib/HDL Operations/Bit Slice  lidx=2  ridx=2
  Bit Slice6 : hdlsllib/HDL Operations/Bit Slice  lidx=1  ridx=1
  Bit Slice7 : hdlsllib/HDL Operations/Bit Slice  lidx=0  ridx=0
  Data Type Conversion{,1..7} (8 alike) : DataTypeConversion  OutDataTypeStr=boolean
  Y0 : Outport  OutDataTypeStr=boolean  SampleTime=1
  Y1 : Outport  Port=2  OutDataTypeStr=boolean  SampleTime=1
  Y2 : Outport  Port=3  OutDataTypeStr=boolean  SampleTime=1
  Y3 : Outport  Port=4  OutDataTypeStr=boolean  SampleTime=1
  Y4 : Outport  Port=5  OutDataTypeStr=boolean  SampleTime=1
  Y5 : Outport  Port=6  OutDataTypeStr=boolean  SampleTime=1
  Y6 : Outport  Port=7  OutDataTypeStr=boolean  SampleTime=1
  Y7 : Outport  Port=8  OutDataTypeStr=boolean  SampleTime=1
  wires:
  X/1 -> Bit Slice4/1, Bit Slice5/1, Bit Slice6/1, Bit Slice7/1, Bit Slice3/1, Bit Slice2/1, Bit Slice1/1, Bit Slice/1
  Data Type Conversion/1 -> Y7/1
  Data Type Conversion1/1 -> Y6/1
  Bit Slice2/1 -> Data Type Conversion2/1
  Bit Slice3/1 -> Data Type Conversion3/1
  Bit Slice4/1 -> Data Type Conversion4/1
  Data Type Conversion6/1 -> Y1/1
  Bit Slice/1 -> Data Type Conversion/1
  Bit Slice1/1 -> Data Type Conversion1/1
  Bit Slice6/1 -> Data Type Conversion6/1
  Data Type Conversion7/1 -> Y0/1
  Bit Slice7/1 -> Data Type Conversion7/1
  Bit Slice5/1 -> Data Type Conversion5/1
  Data Type Conversion2/1 -> Y5/1
  Data Type Conversion3/1 -> Y4/1
  Data Type Conversion4/1 -> Y3/1
  Data Type Conversion5/1 -> Y2/1

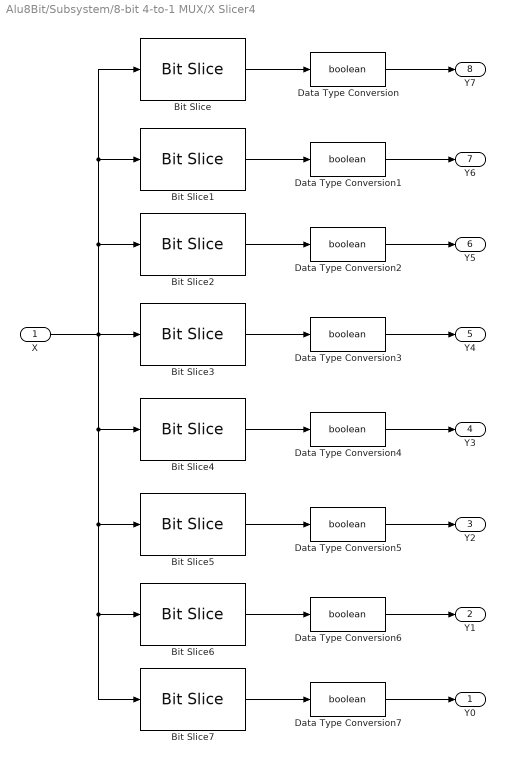
== system Alu8Bit/Subsystem/8-bit 4-to-1 MUX/X Slicer4 ==
  X : Inport  OutDataTypeStr=uint8  SampleTime=1
  Bit Slice : hdlsllib/HDL Operations/Bit Slice  lidx=7  ridx=7
  Bit Slice1 : hdlsllib/HDL Operations/Bit Slice  lidx=6  ridx=6
  Bit Slice2 : hdlsllib/HDL Operations/Bit Slice  lidx=5  ridx=5
  Bit Slice3 : hdlsllib/HDL Operations/Bit Slice  lidx=4  ridx=4
  Bit Slice4 : hdlsllib/HDL Operations/Bit Slice  lidx=3  ridx=3
  Bit Slice5 : hdlsllib/HDL Operations/Bit Slice  lidx=2  ridx=2
  Bit Slice6 : hdlsllib/HDL Operations/Bit Slice  lidx=1  ridx=1
  Bit Slice7 : hdlsllib/HDL Operations/Bit Slice  lidx=0  ridx=0
  Data Type Conversion{,1..7} (8 alike) : DataTypeConversion  OutDataTypeStr=boolean
  Y0 : Outport  OutDataTypeStr=boolean  SampleTime=1
  Y1 : Outport  Port=2  OutDataTypeStr=boolean  SampleTime=1
  Y2 : Outport  Port=3  OutDataTypeStr=boolean  SampleTime=1
  Y3 : Outport  Port=4  OutDataTypeStr=boolean  SampleTime=1
  Y4 : Outport  Port=5  OutDataTypeStr=boolean  SampleTime=1
  Y5 : Outport  Port=6  OutDataTypeStr=boolean  SampleTime=1
  Y6 : Outport  Port=7  OutDataTypeStr=boolean  SampleTime=1
  Y7 : Outport  Port=8  OutDataTypeStr=boolean  SampleTime=1
  wires:
  X/1 -> Bit Slice4/1, Bit Slice5/1, Bit Slice6/1, Bit Slice7/1, Bit Slice3/1, Bit Slice2/1, Bit Slice1/1, Bit Slice/1
  Data Type Conversion/1 -> Y7/1
  Data Type Conversion1/1 -> Y6/1
  Bit Slice2/1 -> Data Type Conversion2/1
  Bit Slice3/1 -> Data Type Conversion3/1
  Bit Slice4/1 -> Data Type Conversion4/1
  Data Type Conversion6/1 -> Y1/1
  Bit Slice/1 -> Data Type Conversion/1
  Bit Slice1/1 -> Data Type Conversion1/1
  Bit Slice6/1 -> Data Type Conversion6/1
  Data Type Conversion7/1 -> Y0/1
  Bit Slice7/1 -> Data Type Conversion7/1
  Bit Slice5/1 -> Data Type Conversion5/1
  Data Type Conversion2/1 -> Y5/1
  Data Type Conversion3/1 -> Y4/1
  Data Type Conversion4/1 -> Y3/1
  Data Type Conversion5/1 -> Y2/1

== system Alu8Bit/Subsystem/8-bit 4-to-1 MUX/X Slicer5 ==
  X : Inport  OutDataTypeStr=uint8  SampleTime=1
  Bit Slice6 : hdlsllib/HDL Operations/Bit Slice  lidx=1  ridx=1
  Bit Slice7 : hdlsllib/HDL Operations/Bit Slice  lidx=0  ridx=0
  Data Type Conversion6 : DataTypeConversion  OutDataTypeStr=boolean
  Data Type Conversion7 : DataTypeConversion  OutDataTypeStr=boolean
  C1 : Outport  OutDataTypeStr=boolean  SampleTime=1
  C2 : Outport  Port=2  OutDataTypeStr=boolean  SampleTime=1
  wires:
  X/1 -> Bit Slice6/1, Bit Slice7/1
  Data Type Conversion6/1 -> C2/1
  Bit Slice6/1 -> Data Type Conversion6/1
  Data Type Conversion7/1 -> C1/1
  Bit Slice7/1 -> Data Type Conversion7/1

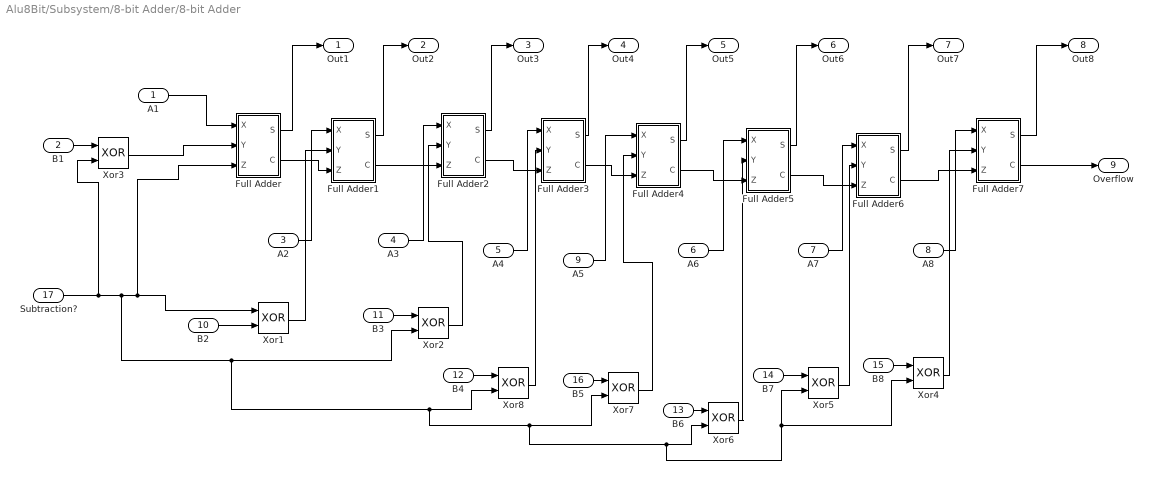
== system Alu8Bit/Subsystem/8-bit Adder/8-bit Adder ==
  A1 : Inport
  B1 : Inport  Port=2
  A2 : Inport  Port=3
  A3 : Inport  Port=4
  A4 : Inport  Port=5
  A6 : Inport  Port=6
  A7 : Inport  Port=7
  A8 : Inport  Port=8
  A5 : Inport  Port=9
  B2 : Inport  Port=10
  B3 : Inport  Port=11
  B4 : Inport  Port=12
  B6 : Inport  Port=13
  B7 : Inport  Port=14
  B8 : Inport  Port=15
  B5 : Inport  Port=16
  Subtraction? : Inport  Port=17  OutDataTypeStr=boolean
  Full Adder : Subsystem
  Full Adder1 : Subsystem
  Full Adder2 : Subsystem
  Full Adder3 : Subsystem
  Full Adder4 : Subsystem
  Full Adder5 : Subsystem
  Full Adder6 : Subsystem
  Full Adder7 : Subsystem
  Xor{1..8} (8 alike) : Logic  Operator=XOR  AllPortsSameDT=off  OutDataTypeStr=boolean
  Out1 : Outport  OutDataTypeStr=boolean
  Out2 : Outport  Port=2  OutDataTypeStr=boolean
  Out3 : Outport  Port=3  OutDataTypeStr=boolean
  Out4 : Outport  Port=4  OutDataTypeStr=boolean
  Out5 : Outport  Port=5  OutDataTypeStr=boolean
  Out6 : Outport  Port=6  OutDataTypeStr=boolean
  Out7 : Outport  Port=7  OutDataTypeStr=boolean
  Out8 : Outport  Port=8  OutDataTypeStr=boolean
  Overflow : Outport  Port=9  OutDataTypeStr=boolean
  wires:
  Full Adder7/2(C) -> Overflow/1
  Full Adder5/2(C) -> Full Adder6/3(Z)
  Full Adder7/1(S) -> Out8/1
  Full Adder4/2(C) -> Full Adder5/3(Z)
  Full Adder/2(C) -> Full Adder1/3(Z)
  Full Adder6/2(C) -> Full Adder7/3(Z)
  Full Adder6/1(S) -> Out7/1
  Full Adder2/2(C) -> Full Adder3/3(Z)
  Full Adder4/1(S) -> Out5/1
  A2/1 -> Full Adder1/1(X)
  A5/1 -> Full Adder4/1(X)
  Full Adder1/1(S) -> Out2/1
  A7/1 -> Full Adder6/1(X)
  Full Adder5/1(S) -> Out6/1
  A1/1 -> Full Adder/1(X)
  A8/1 -> Full Adder7/1(X)
  A6/1 -> Full Adder5/1(X)
  A4/1 -> Full Adder3/1(X)
  Full Adder3/1(S) -> Out4/1
  Full Adder/1(S) -> Out1/1
  Full Adder1/2(C) -> Full Adder2/3(Z)
  A3/1 -> Full Adder2/1(X)
  Full Adder3/2(C) -> Full Adder4/3(Z)
  Full Adder2/1(S) -> Out3/1
  B2/1 -> Xor1/2
  Subtraction?/1 -> Xor3/2, Xor4/2, Xor5/2, Xor6/2, Xor7/2, Xor8/2, Xor2/2, Full Adder/3(Z), Xor1/1
  Xor1/1 -> Full Adder1/2(Y)
  Xor2/1 -> Full Adder2/2(Y)
  B3/1 -> Xor2/1
  B4/1 -> Xor8/1
  Xor8/1 -> Full Adder3/2(Y)
  B5/1 -> Xor7/1
  Xor7/1 -> Full Adder4/2(Y)
  B6/1 -> Xor6/1
  Xor6/1 -> Full Adder5/2(Y)
  B7/1 -> Xor5/1
  Xor5/1 -> Full Adder6/2(Y)
  Xor4/1 -> Full Adder7/2(Y)
  B8/1 -> Xor4/1
  Xor3/1 -> Full Adder/2(Y)
  B1/1 -> Xor3/1

== system Alu8Bit/Subsystem/8-bit Adder/Bit Concat ==
  In1 : Inport
  In2 : Inport  Port=2
  In3 : Inport  Port=3
  In4 : Inport  Port=4
  In5 : Inport  Port=5
  In6 : Inport  Port=6
  In7 : Inport  Port=7
  In8 : Inport  Port=8
  Bit Concat : hdlsllib/HDL Operations/Bit Concat  numInputs=8
  Data Type Conversion : DataTypeConversion  OutDataTypeStr=uint8
  Out1 : Outport
  wires:
  Data Type Conversion/1 -> Out1/1
  In1/1 -> Bit Concat/1
  In4/1 -> Bit Concat/4
  In2/1 -> Bit Concat/2
  In3/1 -> Bit Concat/3
  In5/1 -> Bit Concat/5
  In6/1 -> Bit Concat/6
  In7/1 -> Bit Concat/7
  In8/1 -> Bit Concat/8
  Bit Concat/1 -> Data Type Conversion/1

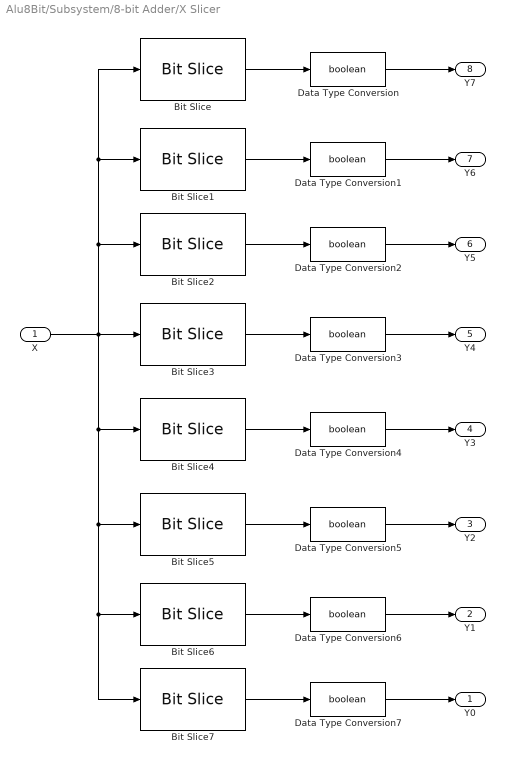
== system Alu8Bit/Subsystem/8-bit Adder/X Slicer ==
  X : Inport  OutDataTypeStr=uint8  SampleTime=1
  Bit Slice : hdlsllib/HDL Operations/Bit Slice  lidx=7  ridx=7
  Bit Slice1 : hdlsllib/HDL Operations/Bit Slice  lidx=6  ridx=6
  Bit Slice2 : hdlsllib/HDL Operations/Bit Slice  lidx=5  ridx=5
  Bit Slice3 : hdlsllib/HDL Operations/Bit Slice  lidx=4  ridx=4
  Bit Slice4 : hdlsllib/HDL Operations/Bit Slice  lidx=3  ridx=3
  Bit Slice5 : hdlsllib/HDL Operations/Bit Slice  lidx=2  ridx=2
  Bit Slice6 : hdlsllib/HDL Operations/Bit Slice  lidx=1  ridx=1
  Bit Slice7 : hdlsllib/HDL Operations/Bit Slice  lidx=0  ridx=0
  Data Type Conversion{,1..7} (8 alike) : DataTypeConversion  OutDataTypeStr=boolean
  Y0 : Outport
  Y1 : Outport  Port=2
  Y2 : Outport  Port=3
  Y3 : Outport  Port=4
  Y4 : Outport  Port=5
  Y5 : Outport  Port=6
  Y6 : Outport  Port=7
  Y7 : Outport  Port=8
  wires:
  X/1 -> Bit Slice4/1, Bit Slice5/1, Bit Slice6/1, Bit Slice7/1, Bit Slice3/1, Bit Slice2/1, Bit Slice1/1, Bit Slice/1
  Data Type Conversion/1 -> Y7/1
  Data Type Conversion1/1 -> Y6/1
  Bit Slice2/1 -> Data Type Conversion2/1
  Bit Slice3/1 -> Data Type Conversion3/1
  Bit Slice4/1 -> Data Type Conversion4/1
  Data Type Conversion6/1 -> Y1/1
  Bit Slice/1 -> Data Type Conversion/1
  Bit Slice1/1 -> Data Type Conversion1/1
  Bit Slice6/1 -> Data Type Conversion6/1
  Data Type Conversion7/1 -> Y0/1
  Bit Slice7/1 -> Data Type Conversion7/1
  Bit Slice5/1 -> Data Type Conversion5/1
  Data Type Conversion2/1 -> Y5/1
  Data Type Conversion3/1 -> Y4/1
  Data Type Conversion4/1 -> Y3/1
  Data Type Conversion5/1 -> Y2/1

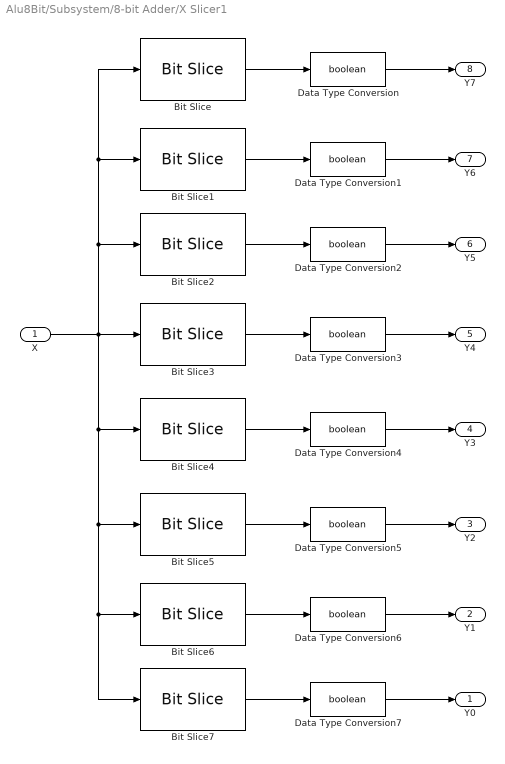
== system Alu8Bit/Subsystem/8-bit Adder/X Slicer1 ==
  X : Inport  OutDataTypeStr=uint8  SampleTime=1
  Bit Slice : hdlsllib/HDL Operations/Bit Slice  lidx=7  ridx=7
  Bit Slice1 : hdlsllib/HDL Operations/Bit Slice  lidx=6  ridx=6
  Bit Slice2 : hdlsllib/HDL Operations/Bit Slice  lidx=5  ridx=5
  Bit Slice3 : hdlsllib/HDL Operations/Bit Slice  lidx=4  ridx=4
  Bit Slice4 : hdlsllib/HDL Operations/Bit Slice  lidx=3  ridx=3
  Bit Slice5 : hdlsllib/HDL Operations/Bit Slice  lidx=2  ridx=2
  Bit Slice6 : hdlsllib/HDL Operations/Bit Slice  lidx=1  ridx=1
  Bit Slice7 : hdlsllib/HDL Operations/Bit Slice  lidx=0  ridx=0
  Data Type Conversion{,1..7} (8 alike) : DataTypeConversion  OutDataTypeStr=boolean
  Y0 : Outport
  Y1 : Outport  Port=2
  Y2 : Outport  Port=3
  Y3 : Outport  Port=4
  Y4 : Outport  Port=5
  Y5 : Outport  Port=6
  Y6 : Outport  Port=7
  Y7 : Outport  Port=8
  wires:
  X/1 -> Bit Slice4/1, Bit Slice5/1, Bit Slice6/1, Bit Slice7/1, Bit Slice3/1, Bit Slice2/1, Bit Slice1/1, Bit Slice/1
  Data Type Conversion/1 -> Y7/1
  Data Type Conversion1/1 -> Y6/1
  Bit Slice2/1 -> Data Type Conversion2/1
  Bit Slice3/1 -> Data Type Conversion3/1
  Bit Slice4/1 -> Data Type Conversion4/1
  Data Type Conversion6/1 -> Y1/1
  Bit Slice/1 -> Data Type Conversion/1
  Bit Slice1/1 -> Data Type Conversion1/1
  Bit Slice6/1 -> Data Type Conversion6/1
  Data Type Conversion7/1 -> Y0/1
  Bit Slice7/1 -> Data Type Conversion7/1
  Bit Slice5/1 -> Data Type Conversion5/1
  Data Type Conversion2/1 -> Y5/1
  Data Type Conversion3/1 -> Y4/1
  Data Type Conversion4/1 -> Y3/1
  Data Type Conversion5/1 -> Y2/1

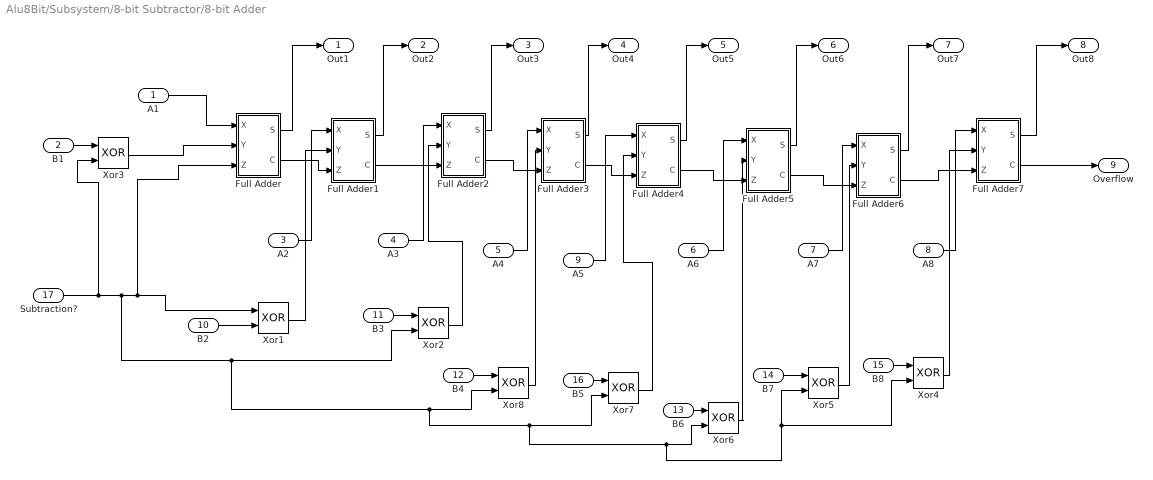
== system Alu8Bit/Subsystem/8-bit Subtractor/8-bit Adder ==
  A1 : Inport
  B1 : Inport  Port=2
  A2 : Inport  Port=3
  A3 : Inport  Port=4
  A4 : Inport  Port=5
  A6 : Inport  Port=6
  A7 : Inport  Port=7
  A8 : Inport  Port=8
  A5 : Inport  Port=9
  B2 : Inport  Port=10
  B3 : Inport  Port=11
  B4 : Inport  Port=12
  B6 : Inport  Port=13
  B7 : Inport  Port=14
  B8 : Inport  Port=15
  B5 : Inport  Port=16
  Subtraction? : Inport  Port=17  OutDataTypeStr=boolean
  Full Adder : Subsystem
  Full Adder1 : Subsystem
  Full Adder2 : Subsystem
  Full Adder3 : Subsystem
  Full Adder4 : Subsystem
  Full Adder5 : Subsystem
  Full Adder6 : Subsystem
  Full Adder7 : Subsystem
  Xor{1..8} (8 alike) : Logic  Operator=XOR  AllPortsSameDT=off  OutDataTypeStr=boolean
  Out1 : Outport  OutDataTypeStr=boolean
  Out2 : Outport  Port=2  OutDataTypeStr=boolean
  Out3 : Outport  Port=3  OutDataTypeStr=boolean
  Out4 : Outport  Port=4  OutDataTypeStr=boolean
  Out5 : Outport  Port=5  OutDataTypeStr=boolean
  Out6 : Outport  Port=6  OutDataTypeStr=boolean
  Out7 : Outport  Port=7  OutDataTypeStr=boolean
  Out8 : Outport  Port=8  OutDataTypeStr=boolean
  Overflow : Outport  Port=9  OutDataTypeStr=boolean
  wires:
  Full Adder7/2(C) -> Overflow/1
  Full Adder5/2(C) -> Full Adder6/3(Z)
  Full Adder7/1(S) -> Out8/1
  Full Adder4/2(C) -> Full Adder5/3(Z)
  Full Adder/2(C) -> Full Adder1/3(Z)
  Full Adder6/2(C) -> Full Adder7/3(Z)
  Full Adder6/1(S) -> Out7/1
  Full Adder2/2(C) -> Full Adder3/3(Z)
  Full Adder4/1(S) -> Out5/1
  A2/1 -> Full Adder1/1(X)
  A5/1 -> Full Adder4/1(X)
  Full Adder1/1(S) -> Out2/1
  A7/1 -> Full Adder6/1(X)
  Full Adder5/1(S) -> Out6/1
  A1/1 -> Full Adder/1(X)
  A8/1 -> Full Adder7/1(X)
  A6/1 -> Full Adder5/1(X)
  A4/1 -> Full Adder3/1(X)
  Full Adder3/1(S) -> Out4/1
  Full Adder/1(S) -> Out1/1
  Full Adder1/2(C) -> Full Adder2/3(Z)
  A3/1 -> Full Adder2/1(X)
  Full Adder3/2(C) -> Full Adder4/3(Z)
  Full Adder2/1(S) -> Out3/1
  B2/1 -> Xor1/2
  Subtraction?/1 -> Xor3/2, Xor4/2, Xor5/2, Xor6/2, Xor7/2, Xor8/2, Xor2/2, Full Adder/3(Z), Xor1/1
  Xor1/1 -> Full Adder1/2(Y)
  Xor2/1 -> Full Adder2/2(Y)
  B3/1 -> Xor2/1
  B4/1 -> Xor8/1
  Xor8/1 -> Full Adder3/2(Y)
  B5/1 -> Xor7/1
  Xor7/1 -> Full Adder4/2(Y)
  B6/1 -> Xor6/1
  Xor6/1 -> Full Adder5/2(Y)
  B7/1 -> Xor5/1
  Xor5/1 -> Full Adder6/2(Y)
  Xor4/1 -> Full Adder7/2(Y)
  B8/1 -> Xor4/1
  Xor3/1 -> Full Adder/2(Y)
  B1/1 -> Xor3/1

== system Alu8Bit/Subsystem/8-bit Subtractor/Bit Concat ==
  In1 : Inport
  In2 : Inport  Port=2
  In3 : Inport  Port=3
  In4 : Inport  Port=4
  In5 : Inport  Port=5
  In6 : Inport  Port=6
  In7 : Inport  Port=7
  In8 : Inport  Port=8
  Bit Concat : hdlsllib/HDL Operations/Bit Concat  numInputs=8
  Data Type Conversion : DataTypeConversion  OutDataTypeStr=uint8
  Out1 : Outport
  wires:
  Data Type Conversion/1 -> Out1/1
  In1/1 -> Bit Concat/1
  In4/1 -> Bit Concat/4
  In2/1 -> Bit Concat/2
  In3/1 -> Bit Concat/3
  In5/1 -> Bit Concat/5
  In6/1 -> Bit Concat/6
  In7/1 -> Bit Concat/7
  In8/1 -> Bit Concat/8
  Bit Concat/1 -> Data Type Conversion/1

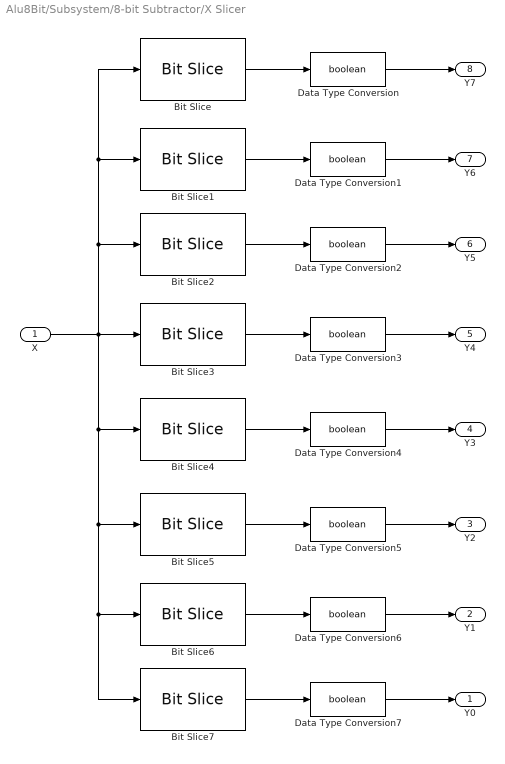
== system Alu8Bit/Subsystem/8-bit Subtractor/X Slicer ==
  X : Inport  OutDataTypeStr=uint8  SampleTime=1
  Bit Slice : hdlsllib/HDL Operations/Bit Slice  lidx=7  ridx=7
  Bit Slice1 : hdlsllib/HDL Operations/Bit Slice  lidx=6  ridx=6
  Bit Slice2 : hdlsllib/HDL Operations/Bit Slice  lidx=5  ridx=5
  Bit Slice3 : hdlsllib/HDL Operations/Bit Slice  lidx=4  ridx=4
  Bit Slice4 : hdlsllib/HDL Operations/Bit Slice  lidx=3  ridx=3
  Bit Slice5 : hdlsllib/HDL Operations/Bit Slice  lidx=2  ridx=2
  Bit Slice6 : hdlsllib/HDL Operations/Bit Slice  lidx=1  ridx=1
  Bit Slice7 : hdlsllib/HDL Operations/Bit Slice  lidx=0  ridx=0
  Data Type Conversion{,1..7} (8 alike) : DataTypeConversion  OutDataTypeStr=boolean
  Y0 : Outport
  Y1 : Outport  Port=2
  Y2 : Outport  Port=3
  Y3 : Outport  Port=4
  Y4 : Outport  Port=5
  Y5 : Outport  Port=6
  Y6 : Outport  Port=7
  Y7 : Outport  Port=8
  wires:
  X/1 -> Bit Slice4/1, Bit Slice5/1, Bit Slice6/1, Bit Slice7/1, Bit Slice3/1, Bit Slice2/1, Bit Slice1/1, Bit Slice/1
  Data Type Conversion/1 -> Y7/1
  Data Type Conversion1/1 -> Y6/1
  Bit Slice2/1 -> Data Type Conversion2/1
  Bit Slice3/1 -> Data Type Conversion3/1
  Bit Slice4/1 -> Data Type Conversion4/1
  Data Type Conversion6/1 -> Y1/1
  Bit Slice/1 -> Data Type Conversion/1
  Bit Slice1/1 -> Data Type Conversion1/1
  Bit Slice6/1 -> Data Type Conversion6/1
  Data Type Conversion7/1 -> Y0/1
  Bit Slice7/1 -> Data Type Conversion7/1
  Bit Slice5/1 -> Data Type Conversion5/1
  Data Type Conversion2/1 -> Y5/1
  Data Type Conversion3/1 -> Y4/1
  Data Type Conversion4/1 -> Y3/1
  Data Type Conversion5/1 -> Y2/1

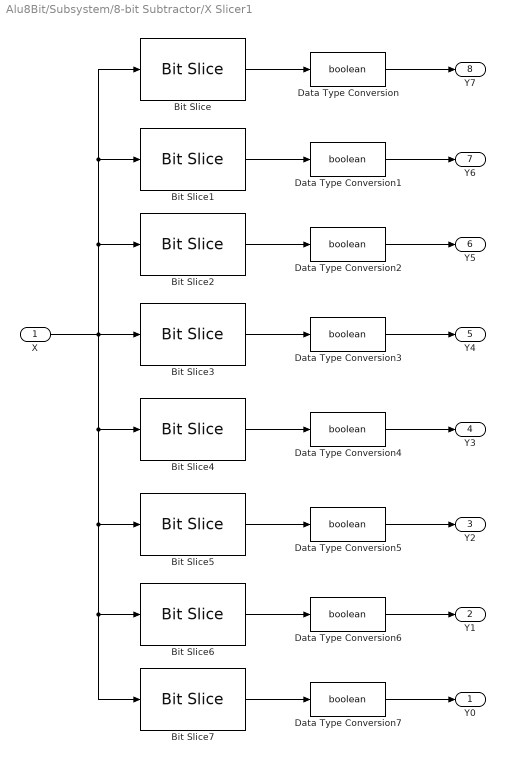
== system Alu8Bit/Subsystem/8-bit Subtractor/X Slicer1 ==
  X : Inport  OutDataTypeStr=uint8  SampleTime=1
  Bit Slice : hdlsllib/HDL Operations/Bit Slice  lidx=7  ridx=7
  Bit Slice1 : hdlsllib/HDL Operations/Bit Slice  lidx=6  ridx=6
  Bit Slice2 : hdlsllib/HDL Operations/Bit Slice  lidx=5  ridx=5
  Bit Slice3 : hdlsllib/HDL Operations/Bit Slice  lidx=4  ridx=4
  Bit Slice4 : hdlsllib/HDL Operations/Bit Slice  lidx=3  ridx=3
  Bit Slice5 : hdlsllib/HDL Operations/Bit Slice  lidx=2  ridx=2
  Bit Slice6 : hdlsllib/HDL Operations/Bit Slice  lidx=1  ridx=1
  Bit Slice7 : hdlsllib/HDL Operations/Bit Slice  lidx=0  ridx=0
  Data Type Conversion{,1..7} (8 alike) : DataTypeConversion  OutDataTypeStr=boolean
  Y0 : Outport
  Y1 : Outport  Port=2
  Y2 : Outport  Port=3
  Y3 : Outport  Port=4
  Y4 : Outport  Port=5
  Y5 : Outport  Port=6
  Y6 : Outport  Port=7
  Y7 : Outport  Port=8
  wires:
  X/1 -> Bit Slice4/1, Bit Slice5/1, Bit Slice6/1, Bit Slice7/1, Bit Slice3/1, Bit Slice2/1, Bit Slice1/1, Bit Slice/1
  Data Type Conversion/1 -> Y7/1
  Data Type Conversion1/1 -> Y6/1
  Bit Slice2/1 -> Data Type Conversion2/1
  Bit Slice3/1 -> Data Type Conversion3/1
  Bit Slice4/1 -> Data Type Conversion4/1
  Data Type Conversion6/1 -> Y1/1
  Bit Slice/1 -> Data Type Conversion/1
  Bit Slice1/1 -> Data Type Conversion1/1
  Bit Slice6/1 -> Data Type Conversion6/1
  Data Type Conversion7/1 -> Y0/1
  Bit Slice7/1 -> Data Type Conversion7/1
  Bit Slice5/1 -> Data Type Conversion5/1
  Data Type Conversion2/1 -> Y5/1
  Data Type Conversion3/1 -> Y4/1
  Data Type Conversion4/1 -> Y3/1
  Data Type Conversion5/1 -> Y2/1

== system Alu8Bit/Subsystem/BitwiseAnd/Bit Concat ==
  In1 : Inport
  In2 : Inport  Port=2
  In3 : Inport  Port=3
  In4 : Inport  Port=4
  In5 : Inport  Port=5
  In6 : Inport  Port=6
  In7 : Inport  Port=7
  In8 : Inport  Port=8
  Bit Concat : hdlsllib/HDL Operations/Bit Concat  numInputs=8
  Data Type Conversion : DataTypeConversion  OutDataTypeStr=uint8
  Out1 : Outport
  wires:
  Data Type Conversion/1 -> Out1/1
  Bit Concat/1 -> Data Type Conversion/1
  In7/1 -> Bit Concat/7
  In1/1 -> Bit Concat/1
  In8/1 -> Bit Concat/8
  In6/1 -> Bit Concat/6
  In2/1 -> Bit Concat/2
  In5/1 -> Bit Concat/5
  In3/1 -> Bit Concat/3
  In4/1 -> Bit Concat/4

== system Alu8Bit/Subsystem/BitwiseAnd/X Slicer1 ==
  X : Inport  OutDataTypeStr=uint8  SampleTime=1
  Bit Slice : hdlsllib/HDL Operations/Bit Slice  lidx=7  ridx=7
  Bit Slice1 : hdlsllib/HDL Operations/Bit Slice  lidx=6  ridx=6
  Bit Slice2 : hdlsllib/HDL Operations/Bit Slice  lidx=5  ridx=5
  Bit Slice3 : hdlsllib/HDL Operations/Bit Slice  lidx=4  ridx=4
  Bit Slice4 : hdlsllib/HDL Operations/Bit Slice  lidx=3  ridx=3
  Bit Slice5 : hdlsllib/HDL Operations/Bit Slice  lidx=2  ridx=2
  Bit Slice6 : hdlsllib/HDL Operations/Bit Slice  lidx=1  ridx=1
  Bit Slice7 : hdlsllib/HDL Operations/Bit Slice  lidx=0  ridx=0
  Data Type Conversion{,1..7} (8 alike) : DataTypeConversion  OutDataTypeStr=boolean
  Y0 : Outport  OutDataTypeStr=boolean  SampleTime=1
  Y1 : Outport  Port=2  OutDataTypeStr=boolean  SampleTime=1
  Y2 : Outport  Port=3  OutDataTypeStr=boolean  SampleTime=1
  Y3 : Outport  Port=4  OutDataTypeStr=boolean  SampleTime=1
  Y4 : Outport  Port=5  OutDataTypeStr=boolean  SampleTime=1
  Y5 : Outport  Port=6  OutDataTypeStr=boolean  SampleTime=1
  Y6 : Outport  Port=7  OutDataTypeStr=boolean  SampleTime=1
  Y7 : Outport  Port=8  OutDataTypeStr=boolean  SampleTime=1
  wires:
  X/1 -> Bit Slice4/1, Bit Slice5/1, Bit Slice6/1, Bit Slice7/1, Bit Slice3/1, Bit Slice2/1, Bit Slice1/1, Bit Slice/1
  Data Type Conversion/1 -> Y7/1
  Data Type Conversion1/1 -> Y6/1
  Bit Slice2/1 -> Data Type Conversion2/1
  Bit Slice3/1 -> Data Type Conversion3/1
  Bit Slice4/1 -> Data Type Conversion4/1
  Data Type Conversion6/1 -> Y1/1
  Bit Slice/1 -> Data Type Conversion/1
  Bit Slice1/1 -> Data Type Conversion1/1
  Bit Slice6/1 -> Data Type Conversion6/1
  Data Type Conversion7/1 -> Y0/1
  Bit Slice7/1 -> Data Type Conversion7/1
  Bit Slice5/1 -> Data Type Conversion5/1
  Data Type Conversion2/1 -> Y5/1
  Data Type Conversion3/1 -> Y4/1
  Data Type Conversion4/1 -> Y3/1
  Data Type Conversion5/1 -> Y2/1
